simulink model "sim1t"  (Simulink 6.0)
settings: Solver=ode45  StartTime=0.0  StopTime=30.0  RelTol=1e-3
settings Model: LastModifiedBy=Administrador
settings DataIOCC: SignalLoggingName=sigsOut
settings DebuggingCC: SolverPrmCheckMsg=none
settings HardwareCC: TargetUnknown=on

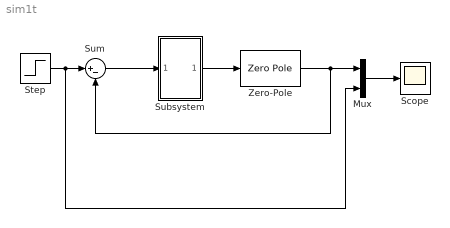
== system sim1t ==
  Mux : Mux  Inputs=2
  Scope : Scope
  Step : Step  Time=0  SampleTime=0
  Subsystem : Subsystem  mask{K1=0.50, K2=0.232, K3=0.3881}
      mask prompts: K1 "Ganho K1 - proporcional"; K2 "Ganho K2 - derivativo"; K3 "Ganho K3 - integral"
  Sum : Sum  Inputs=|+-  SaturateOnIntegerOverflow=on
  Zero-Pole : ZeroPole  Zeros=[]  Poles=[0 -1 -5]  Gain=[60]
  wires:
  Step/1 -> Sum/1, Mux/2
  Sum/1 -> Subsystem/1(In1)
  Subsystem/1(Out1) -> Zero-Pole/1
  Zero-Pole/1 -> Mux/1, Sum/2
  Mux/1 -> Scope/1

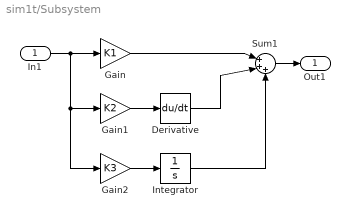
== system sim1t/Subsystem ==
  In1 : Inport  Port=1  LatchInput=off
  Derivative : Derivative
  Gain : Gain  Gain=K1  SaturateOnIntegerOverflow=on
  Gain1 : Gain  Gain=K2  SaturateOnIntegerOverflow=on
  Gain2 : Gain  Gain=K3  SaturateOnIntegerOverflow=on
  Integrator : Integrator
  Sum1 : Sum  Inputs=|+++  SaturateOnIntegerOverflow=on
  Out1 : Outport
  wires:
  Integrator/1 -> Sum1/3
  Derivative/1 -> Sum1/2
  Gain/1 -> Sum1/1
  Gain1/1 -> Derivative/1
  Gain2/1 -> Integrator/1
  In1/1 -> Gain2/1, Gain1/1, Gain/1
  Sum1/1 -> Out1/1
